simulink model "leader_follower_paperli"  (R2020b)
settings: Solver=FixedStepAuto  StartTime=0.0  StopTime=60  FixedStep=0.01  RelTol=1e-3
values from neighbouring files (symbols this model uses):
  A = [-2, 2;-1 1]    [leader_follower_h2.m]    (also in leader_follower_paper_li.m)
  Ak = kron(IN_1,A)    [leader_follower_h2.m]    (also in leader_follower_paper_li.m)
  Aw = kron(IN_1,A-G*C1)+kron(L1,B*F)    [leader_follower_h2.m]    (also in leader_follower_paper_li.m = kron(IN_1,A+B*K)+kron(L1,F*C1))
  Bk = kron(IN_1,B)    [leader_follower_h2.m]    (also in leader_follower_paper_li.m)
  Ck1 = kron(IN_1,C1)    [leader_follower_h2.m]    (also in leader_follower_paper_li.m)
  Ck2 = kron(IN_1,C2)    [leader_follower_h2.m]    (also in leader_follower_paper_li.m)
  Dk1 = kron(IN_1,D1)    [leader_follower_h2.m]    (also in leader_follower_paper_li.m)
  Dk2 = kron(IN_1,D2)    [leader_follower_h2.m]    (also in leader_follower_paper_li.m)
  Ek = kron(IN_1,E)    [leader_follower_h2.m]    (also in leader_follower_paper_li.m)
  Fk = kron(IN_1,F)    [leader_follower_h2.m]    (also in leader_follower_paper_li.m = kron(L1,F))
  Kk = kron(IN_1,K)    [leader_follower_paper_li.m]
  Xint = zeros(1,10)    [leader_follower_h2.m]    (also in leader_follower_paper_li.m)
settings Model: Creator=lenovo  LastModifiedBy=lenovo

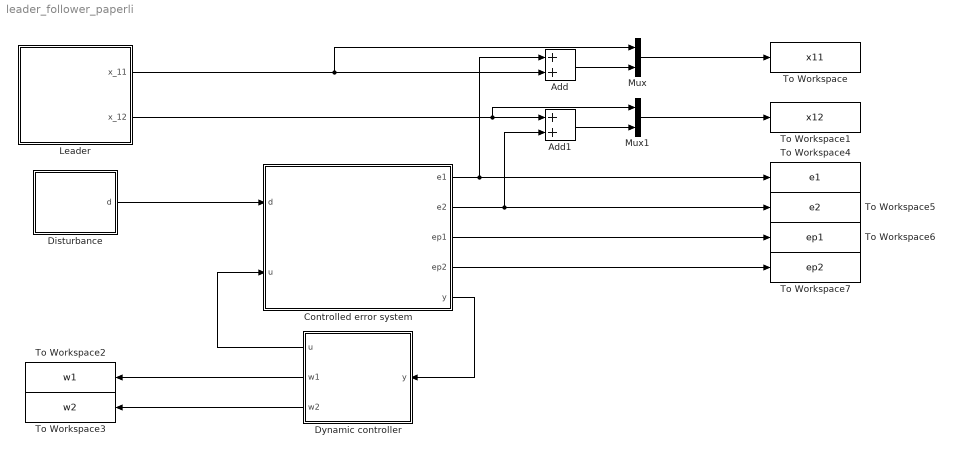
== system leader_follower_paperli ==
  Add : Sum
  Add1 : Sum
  Controlled error system : Subsystem
  Disturbance : Subsystem
  Dynamic controller : Subsystem
  Leader : Subsystem
  Mux : Mux  Inputs=2
  Mux1 : Mux  Inputs=2
  To Workspace : ToWorkspace  VariableName=x11  SampleTime=-1
  To Workspace1 : ToWorkspace  VariableName=x12  SampleTime=-1
  To Workspace2 : ToWorkspace  VariableName=w1  SampleTime=-1
  To Workspace3 : ToWorkspace  VariableName=w2  SampleTime=-1
  To Workspace4 : ToWorkspace  VariableName=e1  SampleTime=-1
  To Workspace5 : ToWorkspace  VariableName=e2  SampleTime=-1
  To Workspace6 : ToWorkspace  VariableName=ep1  SampleTime=-1
  To Workspace7 : ToWorkspace  VariableName=ep2  SampleTime=-1
  wires:
  Dynamic controller/2(w1) -> To Workspace2/1
  Controlled error system/2(e2) -> To Workspace5/1, Add1/2
  Controlled error system/4(ep2) -> To Workspace7/1
  Mux1/1 -> To Workspace1/1
  Dynamic controller/3(w2) -> To Workspace3/1
  Mux/1 -> To Workspace/1
  Add1/1 -> Mux1/2
  Dynamic controller/1(u) -> Controlled error system/2(u)
  Add/1 -> Mux/2
  Controlled error system/1(e1) -> To Workspace4/1, Add/1
  Leader/1(x_11) -> Add/2, Mux/1
  Controlled error system/5(y) -> Dynamic controller/1(y)
  Controlled error system/3(ep1) -> To Workspace6/1
  Leader/2(x_12) -> Mux1/1, Add1/1
  Disturbance/1(d) -> Controlled error system/1(d)

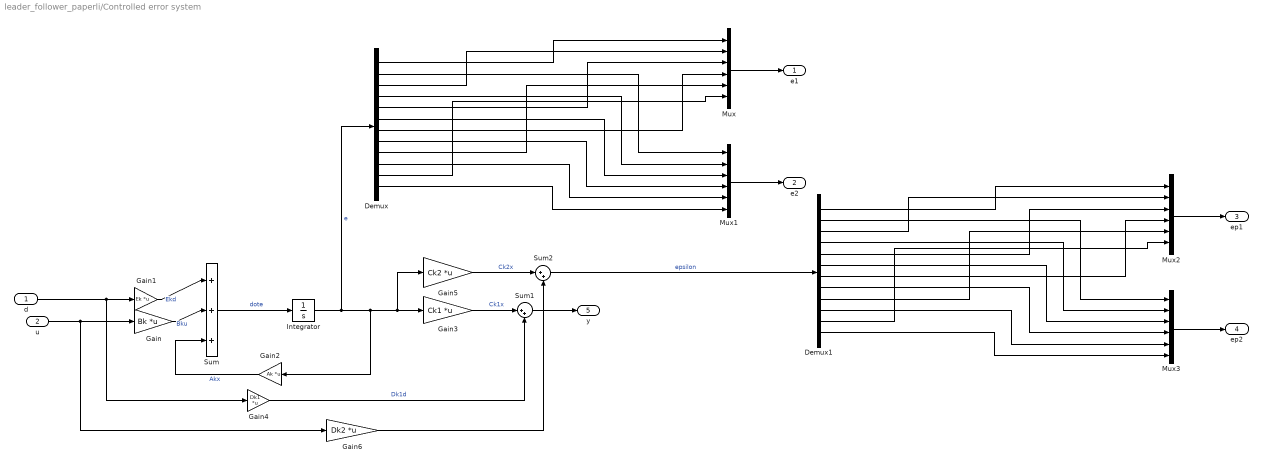
== system leader_follower_paperli/Controlled error system ==
  d : Inport
  u : Inport  Port=2
  Demux : Demux  Outputs=12
  Demux1 : Demux  Outputs=12
  Gain : Gain  Gain=Bk  Multiplication=Matrix(K*u) (u vector)
  Gain1 : Gain  Gain=Ek  Multiplication=Matrix(K*u) (u vector)
  Gain2 : Gain  Gain=Ak  Multiplication=Matrix(K*u) (u vector)
  Gain3 : Gain  Gain=Ck1  Multiplication=Matrix(K*u) (u vector)
  Gain4 : Gain  Gain=Dk1  Multiplication=Matrix(K*u) (u vector)
  Gain5 : Gain  Gain=Ck2  Multiplication=Matrix(K*u) (u vector)
  Gain6 : Gain  Gain=Dk2  Multiplication=Matrix(K*u) (u vector)
  Integrator : Integrator  InitialCondition=Xint
  Mux{,1..3} (4 alike) : Mux  Inputs=6
  Sum : Sum  Inputs=|+++
  Sum1 : Sum  Inputs=|++
  Sum2 : Sum  Inputs=|++
  e1 : Outport
  e2 : Outport  Port=2
  ep1 : Outport  Port=3
  ep2 : Outport  Port=4
  y : Outport  Port=5
  wires:
  Gain3/1 -> Sum1/1  "Ck1x"
  Integrator/1 -> Demux/1, Gain5/1, Gain3/1, Gain2/1  "e"
  Gain5/1 -> Sum2/1  "Ck2x"
  Gain2/1 -> Sum/3  "Akx"
  Sum/1 -> Integrator/1  "dote"
  Gain4/1 -> Sum1/2  "Dk1d"
  Gain1/1 -> Sum/1  "Ekd"
  Gain/1 -> Sum/2  "Bku"
  Sum1/1 -> y/1
  u/1 -> Gain/1, Gain6/1
  Gain6/1 -> Sum2/2
  Mux/1 -> e1/1
  Mux1/1 -> e2/1
  d/1 -> Gain4/1, Gain1/1
  Demux/1 -> Mux/1
  Demux/3 -> Mux/2
  Demux/5 -> Mux/3
  Demux/7 -> Mux/4
  Demux/9 -> Mux/5
  Demux/11 -> Mux/6
  Demux/2 -> Mux1/1
  Demux/4 -> Mux1/2
  Demux/6 -> Mux1/3
  Demux/8 -> Mux1/4
  Demux/10 -> Mux1/5
  Demux/12 -> Mux1/6
  Demux1/11 -> Mux2/6
  Demux1/10 -> Mux3/5
  Demux1/8 -> Mux3/4
  Demux1/3 -> Mux2/2
  Demux1/2 -> Mux3/1
  Demux1/1 -> Mux2/1
  Sum2/1 -> Demux1/1  "epsilon"
  Demux1/7 -> Mux2/4
  Demux1/9 -> Mux2/5
  Demux1/5 -> Mux2/3
  Mux2/1 -> ep1/1
  Demux1/12 -> Mux3/6
  Mux3/1 -> ep2/1
  Demux1/6 -> Mux3/3
  Demux1/4 -> Mux3/2

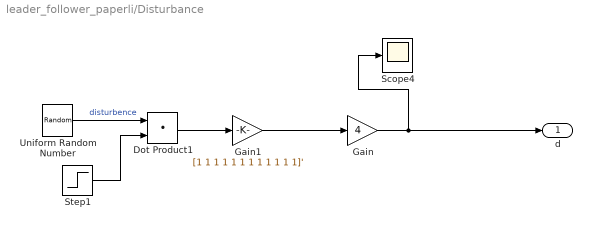
== system leader_follower_paperli/Disturbance ==
  Dot Product1 : DotProduct  InputSameDT=on  OutDataTypeStr=Inherit: Inherit via internal rule
  Gain : Gain  Gain=4
  Gain1 : Gain  Gain=[1 1 1 1 1 1 1 1 1 1 1 1]'
  Scope4 : Scope
  Step1 : Step  Time=100000  Before=1  After=0  SampleTime=0
  Uniform Random Number : UniformRandomNumber  SampleTime=0.1
  d : Outport
  wires:
  Gain/1 -> d/1, Scope4/1
  Dot Product1/1 -> Gain1/1
  Gain1/1 -> Gain/1
  Uniform Random Number/1 -> Dot Product1/1  "disturbence"
  Step1/1 -> Dot Product1/2

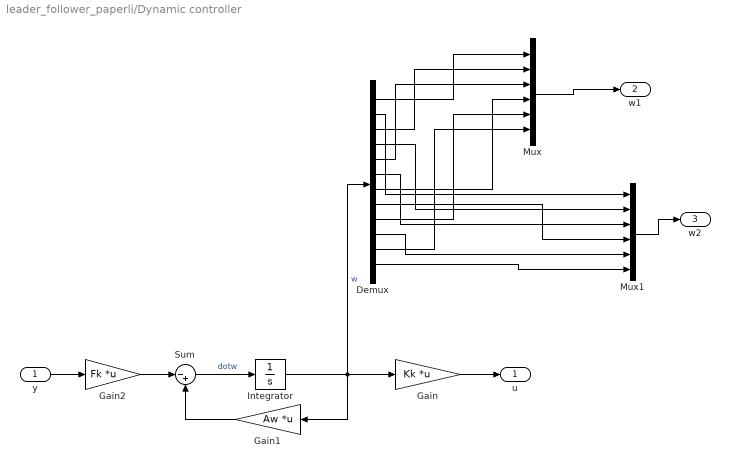
== system leader_follower_paperli/Dynamic controller ==
  y : Inport
  Demux : Demux  Outputs=12
  Gain : Gain  Gain=Kk  Multiplication=Matrix(K*u) (u vector)
  Gain1 : Gain  Gain=Aw  Multiplication=Matrix(K*u) (u vector)
  Gain2 : Gain  Gain=Fk  Multiplication=Matrix(K*u) (u vector)
  Integrator : Integrator
  Mux : Mux  Inputs=6
  Mux1 : Mux  Inputs=6
  Sum : Sum  Inputs=|-+
  u : Outport
  w1 : Outport  Port=2
  w2 : Outport  Port=3
  wires:
  Integrator/1 -> Demux/1, Gain/1, Gain1/1  "w"
  Gain1/1 -> Sum/2
  Gain/1 -> u/1
  y/1 -> Gain2/1
  Sum/1 -> Integrator/1  "dotw"
  Gain2/1 -> Sum/1
  Mux1/1 -> w2/1
  Mux/1 -> w1/1
  Demux/1 -> Mux/1
  Demux/3 -> Mux/2
  Demux/5 -> Mux/3
  Demux/7 -> Mux/4
  Demux/9 -> Mux/5
  Demux/11 -> Mux/6
  Demux/2 -> Mux1/1
  Demux/4 -> Mux1/2
  Demux/6 -> Mux1/3
  Demux/8 -> Mux1/4
  Demux/10 -> Mux1/5
  Demux/12 -> Mux1/6

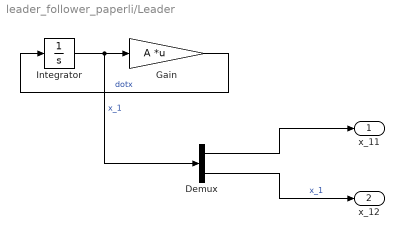
== system leader_follower_paperli/Leader ==
  Demux : Demux  Outputs=2
  Gain : Gain  Gain=A  Multiplication=Matrix(K*u) (u vector)
  Integrator : Integrator  InitialCondition=[2.5,7.5]'
  x_11 : Outport
  x_12 : Outport  Port=2
  wires:
  Gain/1 -> Integrator/1  "dotx"
  Demux/1 -> x_11/1
  Integrator/1 -> Demux/1, Gain/1  "x_1"
  Demux/2 -> x_12/1  "x_1"
